simulink model "test"  (R2021a)
settings: configuration reference "f2_ctrl_config" (kept outside this file)
values from neighbouring files (symbols this model uses):
  sys_regs = 1    [motor_data.sldd]
undefined symbols (not defined in the file or in its folder): btn, com, rmt
settings Model: DataDictionary=motor_data.sldd  Creator=Litao  LastModifiedBy=Litao
settings ConfigSetRef: SourceName=f2_ctrl_config

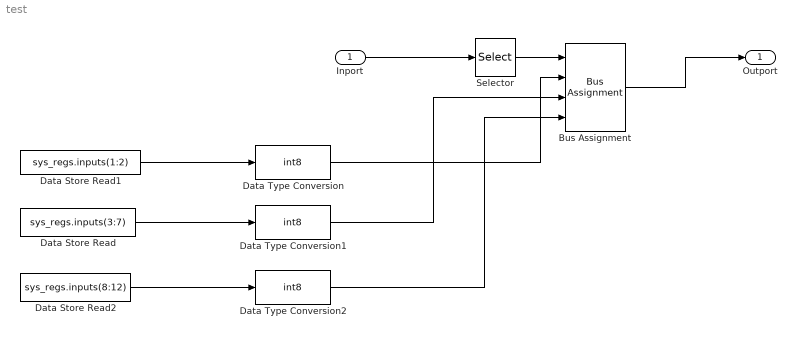
== system test ==
  Inport : Inport  OutDataTypeStr=Bus: ch_signal  PortDimensions=4  Interpolate=off  BusOutputAsStruct=on
  Bus Assignment : BusAssignment  AssignedSignals=btn,com,rmt
  Data Store Read : DataStoreRead  DataStoreName=sys_regs  DataStoreElements=sys_regs.inputs(3:7)  IndexOptions=Index vector (dialog)  Indices=1  OutputSizes=1
  Data Store Read1 : DataStoreRead  DataStoreName=sys_regs  DataStoreElements=sys_regs.inputs(1:2)  IndexOptions=Index vector (dialog)  Indices=1  OutputSizes=1
  Data Store Read2 : DataStoreRead  DataStoreName=sys_regs  DataStoreElements=sys_regs.inputs(8:12)  IndexOptions=Index vector (dialog)  Indices=1  OutputSizes=1
  Data Type Conversion : DataTypeConversion  OutDataTypeStr=int8
  Data Type Conversion1 : DataTypeConversion  OutDataTypeStr=int8
  Data Type Conversion2 : DataTypeConversion  OutDataTypeStr=int8
  Selector : Selector  IndexMode=Zero-based  InputPortWidth=4  IndexOptions=Index vector (dialog)  Indices=[0]  OutputSizes=1
  Outport : Outport
  wires:
  Data Type Conversion/1 -> Bus Assignment/2
  Data Store Read1/1 -> Data Type Conversion/1
  Data Store Read/1 -> Data Type Conversion1/1
  Data Type Conversion1/1 -> Bus Assignment/3
  Data Store Read2/1 -> Data Type Conversion2/1
  Data Type Conversion2/1 -> Bus Assignment/4
  Inport/1 -> Selector/1
  Selector/1 -> Bus Assignment/1
  Bus Assignment/1 -> Outport/1
